simulink model "MultirotorPx4HorizontalThrustOnly"  (R2018b)
settings: Solver=VariableStepAuto  StartTime=0.0  StopTime=10.0  RelTol=1e-3
undefined symbols (not defined in the file): Ctrl
settings Model: Creator=jban039  LastModifiedBy=jeremie

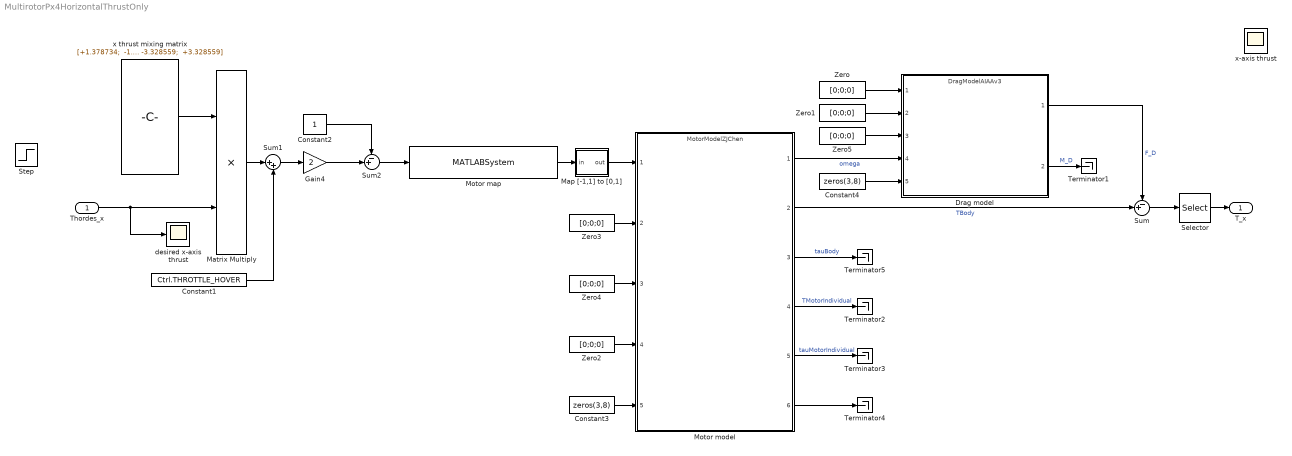
== system MultirotorPx4HorizontalThrustOnly ==
  Thordes_x : Inport
  Constant1 : Constant  Value=Ctrl.THROTTLE_HOVER
  Constant2 : Constant
  Constant3 : Constant  Value=zeros(3,8)
  Constant4 : Constant  Value=zeros(3,8)
  Drag model : ModelReference  ModelNameDialog=DragModelAIAAv3  SimulationMode=Normal  ModelReferenceVersion=1.373
  Gain4 : Gain  Gain=2
  Map [-1,1] to [0,1] : Subsystem
  Matrix Multiply : Product
  Motor map : MATLABSystem  System=MotorMap  airframeConfig=5  SimulateUsing=Code generation
      mask Type: MotorMap
      mask Display:
      | disp(['MOTOR' char(10) 'MAP' char(10) 'octa_x']);
      | port_label('input',1,'px4PWM');
      | port_label('output',1,'simPWM');
  Motor model : ModelReference  ModelNameDialog=MotorModelZJChen  SimulationMode=Normal  ModelReferenceVersion=1.444
  Selector : Selector  InputPortWidth=3  IndexOptions=Index vector (dialog)  Indices=[1]  OutputSizes=1
  Step : Step  After=0.1  SampleTime=0
  Sum : Sum  Inputs=-+|
  Sum1 : Sum  Inputs=|++
  Sum2 : Sum  Inputs=-+|
  Terminator{1..5} (5 alike) : Terminator
  Zero{,1..5} (6 alike) : Constant  Value=[0;0;0]  OutDataTypeStr=Inherit: Inherit via back propagation
  desired x-axis thrust : Scope
  x thrust mixing matrix : Constant  Value=|  VectorParams1D=off
      | [+1.378734;
      |  -1.378734;
      |  -3.328559;
      |  -1.378734;
      |  +1.378734;
      |  +3.328559;
      |  -3.328559;
      |  +3.328559]
  x-axis thrust : Scope
  T_x : Outport
  wires:
  x thrust mixing matrix/1 -> Matrix Multiply/1
  Constant2/1 -> Sum2/1
  Gain4/1 -> Sum2/2
  Matrix Multiply/1 -> Sum1/1
  Map [-1,1] to [0,1]/1(out) -> Motor model/1
  Motor map/1 -> Map [-1,1] to [0,1]/1(in)
  Sum2/1 -> Motor map/1
  Sum1/1 -> Gain4/1
  Constant1/1 -> Sum1/2
  Motor model/1 -> Drag model/4  "omega"
  Drag model/2 -> Terminator1/1  "M_D"
  Drag model/1 -> Sum/1  "F_D"
  Zero/1 -> Drag model/1
  Zero1/1 -> Drag model/2
  Zero2/1 -> Motor model/4
  Constant3/1 -> Motor model/5
  Zero5/1 -> Drag model/3
  Constant4/1 -> Drag model/5
  Zero3/1 -> Motor model/2
  Zero4/1 -> Motor model/3
  Motor model/4 -> Terminator2/1  "TMotorIndividual"
  Motor model/5 -> Terminator3/1  "tauMotorIndividual"
  Motor model/6 -> Terminator4/1
  Motor model/2 -> Sum/2  "TBody"
  Sum/1 -> Selector/1
  Selector/1 -> T_x/1
  Motor model/3 -> Terminator5/1  "tauBody"
  Thordes_x/1 -> desired x-axis thrust/1, Matrix Multiply/2

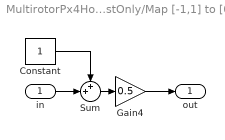
== system MultirotorPx4HorizontalThrustOnly/Map [-1,1] to [0,1] ==
  in : Inport
  Constant : Constant
  Gain4 : Gain  Gain=0.5
  Sum : Sum  Inputs=++|
  out : Outport
  wires:
  Constant/1 -> Sum/1
  in/1 -> Sum/2
  Gain4/1 -> out/1
  Sum/1 -> Gain4/1
